simulink model "BusCreator_nonvirtual"  (R2017b)
settings: Solver=FixedStepDiscrete  StartTime=0.0  StopTime=10.0  FixedStep=0.200000  RelTol=1e-3
PreLoadFcn:
  | % Bus object: subBus
  | clear elems;
  | elems(1) = Simulink.BusElement;
  | elems(1).Name = 'chirp';
  | elems(1).Dimensions = 2;
  | elems(1).DimensionsMode = 'Fixed';
  | elems(1).DataType = 'double';
  | elems(1).SampleTime = -1;
  | elems(1).Complexity = 'real';
  | elems(1).Min = [];
  | elems(1).Max = [];
  | elems(1).DocUnits = '';
  | elems(1).Description = '';
  | 
  | elems(2) = Simulink.BusElement;
  | elems(2).Name = 'sine';
  | elems(2).Dimensions = 3;
  | elems(2).DimensionsMode = 'Fixed';
  | elems(2).DataType = 'int32';
  | elems(2).SampleTime = -1;
  | elems(2).Complexity = 'real';
  | elems(2).Min = [];
  | elems(2).Max = [];
  | elems(2).DocUnits = '';
  | elems(2).Description = '';
  | 
  | subBus = Simulink.Bus;
  | subBus.HeaderFile = '';
  | subBus.Description = '';
  | subBus.DataScope = 'Auto';
  | subBus.Alignment = -1;
  | subBus.Elements = elems;
  | clear elems;
  | assignin('base','subBus', subBus);
  | 
  | % Bus object: topBus
  | clear elems;
  | elems(1) = Simulink.BusElement;
  | elems(1).Name = 'subSignal';
  | elems(1).Dimensions = 1;
  | elems(1).DimensionsMode = 'Fixed';
  | elems(1).DataType = 'Bus: subBus';
  | elems(1).SampleTime = -1;
  | elems(1).Complexity = 'real';
  | elems(1).Min = [];
  | elems(1).Max = [];
  | elems(1).DocUnits = '';
  | elems(1).Description = '';
  | 
  | elems(2) = Simulink.BusElement;
  | elems(2).Name = 'step';
  | elems(2).Dimensions = 4;
  | elems(2).DimensionsMode = 'Fixed';
  | elems(2).DataType = 'boolean';
  | elems(2).SampleTime = -1;
  | elems(2).Complexity = 'real';
  | elems(2).Min = [];
  | elems(2).Max = [];
  | elems(2).DocUnits = '';
  | elems(2).Description = '';
  | 
  | topBus = Simulink.Bus;
  | topBus.HeaderFile = '';
  | topBus.Description = '';
  | topBus.DataScope = 'Auto';
  | topBus.Alignment = -1;
  | topBus.Elements = elems;
  | clear elems;
  | assignin('base','topBus', topBus);
settings Model: Creator=The MathWorks, Inc.  LastModifiedBy=hbourbou
settings OptimizationCC: LifeSpan=inf
settings DebuggingCC: SFExecutionAtInitializationDiag=none
settings HardwareCC: ProdBitPerSizeT=32  ProdBitPerPtrDiffT=32  ProdWordSize=32  ProdHWDeviceType=Specified
settings CodeAppCC: StateflowObjectComments=on
settings ConfigComp: CovMetricSettings=dswe

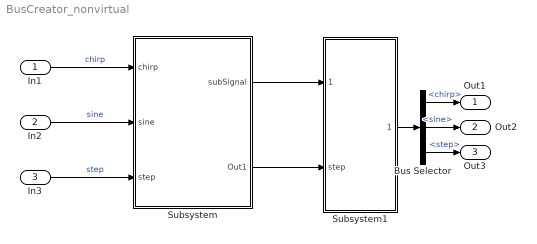
== system BusCreator_nonvirtual ==
  In1 : Inport  PortDimensions=2
  In2 : Inport  Port=2  OutDataTypeStr=int32  PortDimensions=3
  In3 : Inport  Port=3  OutDataTypeStr=boolean  PortDimensions=4
  Bus Selector : BusSelector  OutputSignals=subSignal.chirp,subSignal.sine,step
  Subsystem : Subsystem
  Subsystem1 : Subsystem
  Out1 : Outport
  Out2 : Outport  Port=2
  Out3 : Outport  Port=3
  wires:
  In3/1 -> Subsystem/3(step)  "step"
  In1/1 -> Subsystem/1(chirp)  "chirp"
  In2/1 -> Subsystem/2(sine)  "sine"
  Subsystem/1(subSignal) -> Subsystem1/1(subBus)
  Subsystem/2(Out1) -> Subsystem1/2(step)
  Subsystem1/1(nestedBus) -> Bus Selector/1
  Bus Selector/1 -> Out1/1  "<chirp>"
  Bus Selector/2 -> Out2/1  "<sine>"
  Bus Selector/3 -> Out3/1  "<step>"

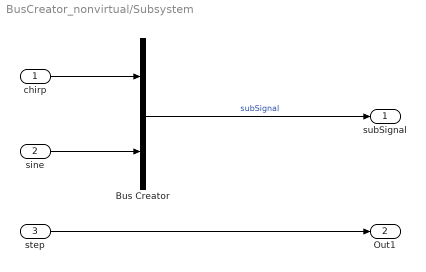
== system BusCreator_nonvirtual/Subsystem ==
  chirp : Inport
  sine : Inport  Port=2
  step : Inport  Port=3  OutDataTypeStr=boolean  PortDimensions=4
  Bus Creator : BusCreator  Inputs=2  OutDataTypeStr=Bus: subBus  NonVirtualBus=on
      settings: AttributesFormatString=SubBus
  subSignal : Outport
  Out1 : Outport  Port=2
  wires:
  Bus Creator/1 -> subSignal/1  "subSignal"
  chirp/1 -> Bus Creator/1
  sine/1 -> Bus Creator/2
  step/1 -> Out1/1

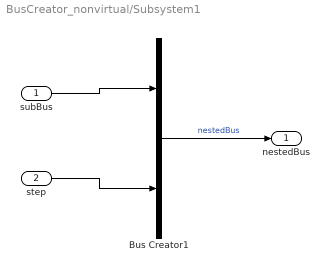
== system BusCreator_nonvirtual/Subsystem1 ==
  subBus : Inport
  step : Inport  Port=2
  Bus Creator1 : BusCreator  Inputs=2  OutDataTypeStr=Bus: topBus  NonVirtualBus=on
      settings: AttributesFormatString=NestedBus
  nestedBus : Outport
  wires:
  subBus/1 -> Bus Creator1/1
  Bus Creator1/1 -> nestedBus/1  "nestedBus"
  step/1 -> Bus Creator1/2
